simulink model "SIMULINK"  (R2022b)
settings: Solver=VariableStepAuto  StartTime=0.0  StopTime=10.0  RelTol=1e-3
libraries: slpidlib x6, robotcorelib x1
settings Model: Creator=kisho  LastModifiedBy=Kishor

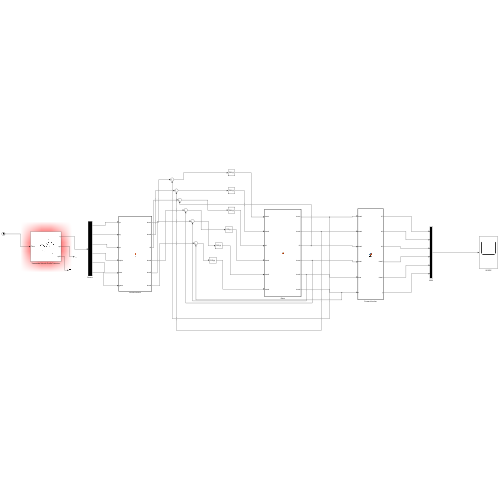
[thumbnail: Simulink's stored preview of the top-level diagram]
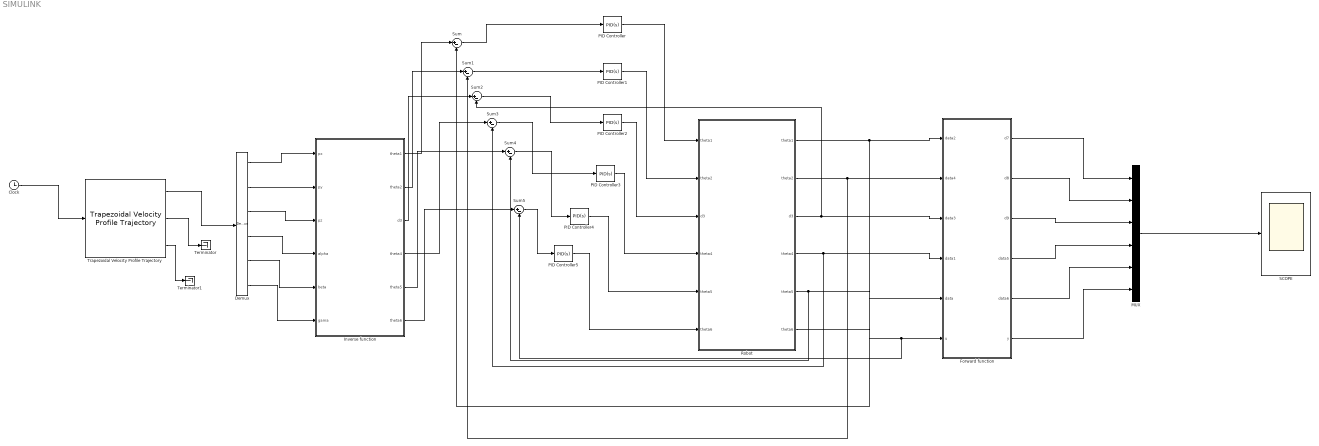
== system SIMULINK ==
  " Robot" : MATLAB Function  TreatAsAtomicUnit=on
  Clock : Clock
  "Demux " : Demux  Outputs=6
  Forward function : MATLAB Function  TreatAsAtomicUnit=on
  Inverse function : MATLAB Function  TreatAsAtomicUnit=on
  MUX : Mux  Inputs=6
  PID Controller{,1..5} (6 alike) : slpidlib/PID Controller  Controller=PID  Form=Parallel  TimeDomain=Continuous-time  UseExternalTs=off  SampleTime=-1  IntegratorMethod=Forward Euler  FilterMethod=Forward Euler  ControllerParametersSource=internal  P=1  I=1  UseKiTs=off  D=0  N=100  UseFilter=on  TunerSelectOption=Transfer Function Based (PID Tuner App)  InitialConditionSource=internal  InitialConditionForIntegrator=0  InitialConditionForFilter=0  DifferentiatorICPrevScaledInput=0  ExternalReset=none  TrackingMode=off  Kt=1  LimitOutput=off  SatLimitsSource=internal  UpperSaturationLimit=inf  LowerSaturationLimit=-inf  LinearizeAsGain=on  AntiWindupMode=none  Kb=1  LimitIntegrator=off  UpperIntegratorSaturationLimit=inf  LowerIntegratorSaturationLimit=-inf  POutMin=[]  POutMax=[]  IOutMin=[]  IOutMax=[]  DOutMin=[]  DOutMax=[]  NOutMin=[]  NOutMax=[]  SumOutMin=[]  SumOutMax=[]  SaturationOutMin=[]  SaturationOutMax=[]  PParamMin=[]  PParamMax=[]  IParamMin=[]  IParamMax=[]  DParamMin=[]  DParamMax=[]  NParamMin=[]  NParamMax=[]  KbParamMin=[]  KbParamMax=[]  KtParamMin=[]  KtParamMax=[]  KbOutMin=[]  KbOutMax=[]  KtOutMin=[]  KtOutMax=[]  IntegratorOutMin=[]  IntegratorOutMax=[]  FilterOutMin=[]  FilterOutMax=[]  SumI1OutMin=[]  SumI1OutMax=[]  SumI2OutMin=[]  SumI2OutMax=[]  SumI3OutMin=[]  SumI3OutMax=[]  SumI4OutMin=[]  SumI4OutMax=[]  SumDOutMin=[]  SumDOutMax=[]  DifferentiatorOutMin=[]  DifferentiatorOutMax=[]  FilterDiffOutCoefMin=[]  FilterDiffOutCoefMax=[]  ReciprocalOutMin=[]  ReciprocalOutMax=[]  SumDenOutMin=[]  SumDenOutMax=[]  SumNumOutMin=[]  SumNumOutMax=[]  DivideOutMin=[]  DivideOutMax=[]  UdiffTsProdOutMin=[]  UdiffTsProdOutMax=[]  NTsProdOutMin=[]  NTsProdOutMax=[]  UintegralTsProdOutMin=[]  UintegralTsProdOutMax=[]  UngainTsProdOutMin=[]  UngainTsProdOutMax=[]  ClampingZeroOutDataTypeStr=Inherit: Inherit via back propagation  ClampingZeroOutMin=[]  ClampingZeroOutMax=[]  FilterDenConstantOutDataTypeStr=Inherit: Inherit via back propagation  FilterDenConstantOutMin=[]  FilterDenConstantOutMax=[]  PCopyOutDataTypeStr=Inherit: Inherit via back propagation  PCopyOutMin=[]  PCopyOutMax=[]  NCopyOutDataTypeStr=Inherit: Inherit via back propagation  NCopyOutMin=[]  NCopyOutMax=[]  IntegratorContinuousStateAttributes=''  IntegratorStateMustResolveToSignalObject=off  IntegratorRTWStateStorageClass=Auto  FilterContinuousStateAttributes=''  FilterStateMustResolveToSignalObject=off  FilterRTWStateStorageClass=Auto  ParallelPVariant=InternalParameters  IdealPVariant=Disabled  IVariant=InternalParameters  DVariant=InternalParameters  IntegratorVariant=Continuous  SatVariant=Disabled  AWVariant=Passthrough  PCopyVariant=Disabled  TRVariant=Disabled  FdbkBlocksVariant=Forward  IdealPFdbkVariant=Disabled  SatFdbkVariant=Disabled  DerivativeFilterVariant=ContFilter  NVariant=InternalParameters  NCopyVariant=Disabled  FilterICVariant=InternalICsFilter  IntegratorICVariant=InternalICs  ExternalResetVariant=Disabled  TRSumVariant=Passthrough  SumFdbkVariant=Disabled  SumVariant=Sum_PID  TsampFilterVariant=InternalTs  TsampNgainVariant=Passthrough  TsampIntegralVariant=Passthrough  ExternalSaturationOutDataTypeStr=Inherit: Same as second input
  SCOPE : Scope
  Sum{,1..5} (6 alike) : Sum  Inputs=|+-
  Terminator : Terminator
  Terminator1 : Terminator
  Trapezoidal Velocity Profile Trajectory : robotcorelib/Trapezoidal Velocity Profile Trajectory  WaypointSource=Internal  Waypoints=wp  NumParams=0  Parameter1=Peak Velocity  Parameter2=End Time  ParameterSource=Internal  PeakVelocity=[ 2; 2 ]  Acceleration=[ 1; 2 ]  EndTime=[ 1; 1 ]  AccelTime=[ 1; 2 ]  SimulateUsing=Interpreted execution
  wires:
  Clock/1 -> Trapezoidal Velocity Profile Trajectory/1
  Trapezoidal Velocity Profile Trajectory/1 -> "Demux "/1
  Inverse function/1(theta1) -> Sum/1
  Inverse function/2(theta2) -> Sum1/1
  Inverse function/3(d3) -> Sum2/1
  Inverse function/4(theta4) -> Sum3/1
  Inverse function/5(theta5) -> Sum4/1
  Inverse function/6(theta6) -> Sum5/1
  " Robot"/1(theta1) -> Forward function/1(data2), Sum/2
  " Robot"/2(theta2) -> Sum1/2, Forward function/2(data4)
  " Robot"/3(d3) -> Forward function/3(data3), Sum2/2
  " Robot"/4(theta4) -> Sum3/2, Forward function/4(data1)
  " Robot"/5(theta5) -> Sum4/2, Forward function/5(data)
  " Robot"/6(theta6) -> Sum5/2, Forward function/6(u)
  "Demux "/1 -> Inverse function/1(px)
  "Demux "/2 -> Inverse function/2(py)
  "Demux "/3 -> Inverse function/3(pz)
  "Demux "/4 -> Inverse function/4(alpha)
  "Demux "/5 -> Inverse function/5(beta)
  "Demux "/6 -> Inverse function/6(gama)
  Forward function/5(data6) -> MUX/5
  Forward function/1(d7) -> MUX/1
  Forward function/2(d8) -> MUX/2
  Forward function/3(d9) -> MUX/3
  Forward function/4(data5) -> MUX/4
  Forward function/6(y) -> MUX/6
  MUX/1 -> SCOPE/1
  PID Controller/1 -> " Robot"/1("theta1 ")
  Sum/1 -> PID Controller/1
  PID Controller1/1 -> " Robot"/2("theta2 ")
  PID Controller2/1 -> " Robot"/3("d3 ")
  PID Controller3/1 -> " Robot"/4("theta4 ")
  PID Controller4/1 -> " Robot"/5("theta5 ")
  PID Controller5/1 -> " Robot"/6("theta6 ")
  Sum1/1 -> PID Controller1/1
  Sum2/1 -> PID Controller2/1
  Sum3/1 -> PID Controller3/1
  Sum4/1 -> PID Controller4/1
  Sum5/1 -> PID Controller5/1
  Trapezoidal Velocity Profile Trajectory/2 -> Terminator/1
  Trapezoidal Velocity Profile Trajectory/3 -> Terminator1/1

== matlab function SIMULINK/Forward function ==
  data: d7 output; d8 output; d9 output; data5 output; data6 output; data2 input; data4 input; data3 input; data1 input; data input; u input; y output
function [d7, d8, d9, data5, data6, y]= fcn(data2, data4, data3, data1, data, u)

 T10 = DHFUNCTION(a0,alpha0,d1,t1*pi/180); 
 T21 = DHFUNCTION(a1,alpha1,d2,(t2-90)*pi/180);  
 T32 = DHFUNCTION(a2,alpha2,d3,0) ;
 T43 = DHFUNCTION(a3,alpha3,d4,t4*pi/180); 
 T54 = DHFUNCTION(a4,alpha4,d5,t5*pi/180); 
 T65 = DHFUNCTION(a5,alpha5,d6,t6*pi/180);

%Once the homogeneous transformation matrix of each link is obtained, forward kinematic chain can be applied to achieve the position and orientation of the robot end-effector with respect to the robot base

T20 = T10*T21; 
T30 = T20*T32; 
T40 = T30*T43; 
T50 = T40*T54; 
T60 = (T50*T65)
% T60 = simplify(T60)

Xw = T60(1,4); 
Yw = T60(2,4); 
Zw = T60(3,4); 
P6 = [Xw;Yw;Zw]

end

== matlab function SIMULINK/Inverse function ==
  data: px input; py input; pz input; alpha input; beta input; gama input; theta1 output; theta2 output; d3 output; theta4 output; theta5 output; theta6 output
function [theta1,theta2, d3, theta4, theta5, theta6] = fcn(px, py, pz, alpha, beta, gama)

coder.extrinsic("INVERSE_KINEMATICS_PROPER")

k =INVERSE_KINEMATICS_PROPER(px, py, pz, alpha, beta, gama)
k

% syms  theta4 theta5 theta6 theta1 theta2 d3;

% px = input("Enter the x coordinate: ");
% py = input("Enter the y coordinate: ");
% pz = input("Enter the z coordinate: ");
% alpha = input('Enter the value of alpha: ');
% beta = input('Enter the value of beta: ');
% gama = input('Enter th value of gama: ');

% theta1 = theta1 * pi/180;
% theta2 = theta2 * pi/180;

% theta4 = theta4 * pi/180;
% theta5 = theta5 * pi/180;
% theta6 = theta6 * pi/180;

% T01 = DHFUNCTION(0,0,200,theta1); %first transformation matrix from base to joint 1
% T12 = DHFUNCTION(70,-pi/2,0,theta2-1.57); %Transfornation matrix from joint 1 to joint 2
% T23 = DHFUNCTION(360,0,d3,0); %Transfornation matrix from joint 2 to joint 3
% T34 = DHFUNCTION(0,-pi/2,380,theta4); %Transfornation matrix from joint 3 to joint 4
% T45 = DHFUNCTION(0,pi/2,0,theta5); %Transfornation matrix from joint 4 to joint 5
% T56 = DHFUNCTION(0,-pi/2,0,theta6); %Transfornation matrix from joint 5 to joint 6
% 
% T60 = T01 * T12 * T23 * T34 * T45 * T56;
% 
% eq1 = px == T60(1,4);
% eq2 = py == T60(2,4);
% eq3 = pz == T60(3,4);
% 
% solution = solve([eq1, eq2, eq3], [theta1, theta2, d3]);
% 
% t1 = solution.theta1;
% t2 = solution.theta2;
% d3 = solution.d3;
% 
% t1 = eval(real(t1))
% t2 = eval(real(t2))
% d3 = eval(real(d3))

== matlab function SIMULINK/ Robot ==
  data: theta1 output; theta2 output; d3 output; theta4 output; theta5 output; theta1 input; theta2 input; d3 input; theta4 input; theta5 input; theta6 input; theta6 output
function [theta1, theta2, d3, theta4, theta5, theta6]= fcn(theta1, theta2, d3, theta4, theta5, theta6)

T01 = DHFUNCTION(0,0,200,theta1); %first transformation matrix from base to joint 1
T12 = DHFUNCTION(70,-pi/2,0,theta2-(pi/2)); %Transfornation matrix from joint 1 to joint 2
T23 = DHFUNCTION(360,0,d3,0); %Transfornation matrix from joint 2 to joint 3
T34 = DHFUNCTION(0,-pi/2,380,theta4); %Transfornation matrix from joint 3 to joint 4
T45 = DHFUNCTION(0,pi/2,0,theta5); %Transfornation matrix from joint 4 to joint 5
T56 = DHFUNCTION(0,-pi/2,0,theta6); %Transfornation matrix from joint 5 to joint 6

T02 = T01*T12; 
T03 = T02*T23; 
T04 = T03*T34; 
T05 = T04*T45; 
T06 = T05*T56;

p0=T01(:,4);
p1=T02(:,4);
p2=T03(:,4);
p3=T04(:,4);
p4=T05(:,4);
p5=T06(:,4);

plotmat = [p0,p1,p2,p3,p4,p5];
plot3(plotmat(1,:), plotmat(2,:), plotmat(3,:));
end
